simulink model "l512_devel_pps"  (R2012b)
settings: Solver=ode45  StartTime=0.0  StopTime=15000  RelTol=1e-3
undefined symbols (not defined in the file): sfp
libraries: xbsIndex_r4 x6414, casper_library_misc x268, casper_library_delays x134, xps_library x12, simulink x1, gavrt_library x1, xbsReplacements_r4 x1
(part 1 of 67)
settings Model: Creator=jkocz  LastModifiedBy=dprice
settings Model: ModifiedComment=|
  | dprice -- Mon Apr 06 20:09:48 2015 -- Version 1.459
  | Compiled successfully
settings Model: ModifiedHistory=|
  | dprice -- Mon Apr 06 20:09:48 2015 -- Version 1.459
  | Compiled successfully
  | 
  | dprice -- Mon Apr 06 16:18:15 2015 -- Version 1.458
  | 
  | Changed pps delay to about 0.1s
  | 
  | dprice -- Fri Mar 13 15:46:33 2015 -- Version 1.457
  | 
  | 
  | dprice -- Fri Mar 13 15:34:50 2015 -- Version 1.456
  | Copied triggering over to f1 - f4
  | 
  | dprice -- Fri Mar 13 15:31:03 2015 -- Version 1.455
  | 
  | Added better triggering of RMS monitor
  | 
  | dprice -- Wed Jan 21 17:17:07 2015 -- Version 1.454
  | 
  | 
  | dprice -- Wed Jan 21 14:02:39 2015 -- Version 1.453
  | changed to be triggered by correct pps
  | 
  | dprice -- Thu Jan 15 16:51:06 2015 -- Version 1.452
  | dropped core back to 200 MHz from 216 MHz
  | 
  | dprice -- Thu Jan 15 13:30:59 2015 -- Version 1.451
  | 
  | Changed to use PPS triggered vacc. Needs testing!
  | 
  | dprice -- Thu Jan 15 13:21:59 2015 -- Version 1.450
  | 
  | 
  | dprice -- Thu Jan 15 13:19:39 2015 -- Version 1.449
  | 
  | 
  | dprice -- Thu Jan 15 13:13:52 2015 -- Version 1.448
  | 
  | Adding pps triggered vacc
  | 
  | dprice -- Tue Jan 13 15:35:09 2015 -- Version 1.447
  | 
  | Updated to spectrometer f_engine core
  | 
  | dprice -- Wed Dec 17 17:14:12 2014 -- Version 1.446
  | 
  | added some snap blocks to do eq0 output rms tests
  | 
  | dprice -- Fri Nov 21 18:19:20 2014 -- Version 1.445
  | 
  | 
  | dprice -- Fri Nov 21 15:29:28 2014 -- Version 1.444
  | 
  | 
  | dprice -- Fri Nov 21 15:28:21 2014 -- Version 1.443
  | 
  | 
  | dprice -- Fri Nov 21 15:22:12 2014 -- Version 1.442
  | 
  | About to try a compile
  | 
  | dprice -- Fri Nov 21 15:19:27 2014 -- Version 1.441
  | 
  | 
  | dprice -- Fri Nov 21 15:10:28 2014 -- Version 1.440
  | 
  | about to crash :/
  | 
  | dprice -- Thu Dec 19 14:05:55 2013 -- Version 1.439
  | 
  | Removed scope blocks in 10GbE spacketizer
  | 
  | dprice -- Thu Dec 12 01:39:04 2013 -- Version 1.438
  | 
  | Moved pfb and eq to black boxes. Hopefully compile times are a little quicker now...
  | 
  | dprice -- Wed Dec 11 11:19:03 2013 -- Version 1.437
  | 
  | Updated coeff generator (cg) with separate sky BRAM for switching (sw_sky), renamed sky to bpass, and changed from 18 bit to 32 bit coefficients
  | 
  | dprice -- Tue Dec 10 14:55:05 2013 -- Version 1.436
  | 
  | Closing session
  | 
  | dprice -- Sat Dec 07 16:46:59 2013 -- Version 1.435
  | Fixed bool slicing on tgbe_en
  | 
  | dprice -- Wed Dec 04 22:02:25 2013 -- Version 1.434
  | 
  | Trying to compile with 4x gbes in the design
  | 
  | dprice -- Wed Dec 04 21:44:55 2013 -- Version 1.433
  | 
  | Added extra tgbe blocks for failover
  | 
  | dprice -- Wed Dec 04 17:45:31 2013 -- Version 1.432
  | 
  | Renamed coeff_gen cg to save on length of bram name
  | 
  | dprice -- Wed Dec 04 17:38:25 2013 -- Version 1.431
  | 
  | Copied logic across to all fft/fX blocks. Trying first compile.
  | 
  | dprice -- Wed Dec 04 17:29:39 2013 -- Version 1.430
  | 
  | Modified eq block to allow selecting between switched and all-sky modes
  | 
  | dprice -- Wed Dec 04 16:56:15 2013 -- Version 1.429
  | 
  | Adding switching assembly coefficient selection by pps
  | 
  | dprice -- Wed Nov 06 11:09:49 2013 -- Version 1.428
  | 
  | Changed back down to 216 MHz. Added a post-eq snap block for testing of equalization levels
  | 
  | dprice -- Tue Nov 05 18:21:00 2013 -- Version 1.427
  | 
  | Removed scopes as they bring up an irritating message each time you try and compile
  | 
  | dprice -- Tue Nov 05 14:30:34 2013 -- Version 1.426
  | 
  | Found timing issues with round block. Added a mask and increased latency in convert and multiply.
  | 
  | dprice -- Tue Nov 05 11:43:26 2013 -- Version 1.423
  | 
  | Changed clock to 239 MHz, just to see if it still compiles...
  | 
  | dprice -- Tue Nov 05 11:43:26 2013 -- Version 1.423
  | 
  | Changed clock to 239 MHz, just to see if it still compiles...
  | 
  | dprice -- Tue Nov 05 09:11:40 2013 -- Version 1.422
  | 
  | Design compiled successfully at 210 MHz using pblock constraints (hstack). Now bumping to 216 MHz.
  | Added status LEDs to design for PPS and TX
  | 
  | dprice -- Mon Nov 04 16:36:08 2013 -- Version 1.421
  | 
  | Added pipeline delays to yelllow block I/O in effort to aid timing. Worst offending net was the rst yellow block, presumably due to fanout.
  | 
  | Also modified the ADC thresholding logic to use a BRAM vector accumulator.
  | 
  | dprice -- Tue Oct 29 13:55:56 2013 -- Version 1.412
  | 
  | Fixed mux error - due to goto tag mismatch
  | 
  | dprice -- Tue Oct 29 13:55:56 2013 -- Version 1.412
  | 
  | Fixed mux error - due to goto tag mismatch
  | 
  | dprice -- Tue Oct 29 11:53:04 2013 -- Version 1.411
  | 
  | WTF is wrong with these mux blocks? Keep getting error on dtype in on muxes in packetbuffer.
  | 
  | dprice -- Mon Oct 28 18:12:23 2013 -- Version 1.410
  | 
  | 
  | dprice -- Mon Oct 28 18:11:25 2013 -- Version 1.409
  | 
  | Need to remove slice on FFT_SHIFTS
  | 
  | * Black boxed FFT
  | * Added ADC overflow logic and snap.
settings DataIOCC: SignalLoggingSaveFormat=ModelDataLogs
settings DebuggingCC: FcnCallInpInsideContextMsg=UseLocalSettings  StrictBusMsg=Warning
settings GRTTargetCC: CombineOutputUpdateFcns=off  GRTInterface=on

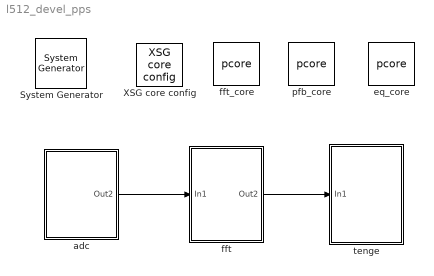
== system l512_devel_pps ==
  " System Generator" : xbsIndex_r4/ System Generator  Tag=genX  xilinxfamily=virtex6  part=xc6vsx475t  speed=-1  package=ff1759  synthesis_tool=XST  clock_wrapper=Clock Enables  directory=./l512_devel_pps/sysgen  proj_type=Project Navigator  Synth_file=XST Defaults  Impl_file=ISE Defaults  testbench=off  simulink_period=1  sysclk_period=5  dcm_input_clock_period=100  incr_netlist=off  trim_vbits=Everywhere in SubSystem  dbl_ovrd=According to Block Masks  core_generation=According to Block Masks  run_coregen=off  deprecated_control=off  eval_field=0  block_type=sysgen
      settings: block_version=11.4
  XSG core config : xps_library/XSG core config  Tag=xps:xsg  hw_sys=ROACH2:sx475t  clk_src=adc0_clk  ROACH_clk_src=adc0_clk  ROACH2_clk_src=adc0_clk  clk_rate=200  sample_period=1  synthesis_tool=XST
  adc : Subsystem
  eq_core : xps_library/pcore  Tag=xps:pcore  pcore_path=/data1/dprice/leda512/bb/eq_basic_core/eq_basic_core.ngc
  fft : Subsystem
  fft_core : xps_library/pcore  Tag=xps:pcore  pcore_path=/data1/dprice/leda512/bb/fft_core/fft_core.ngc
  pfb_core : xps_library/pcore  Tag=xps:pcore  pcore_path=/data1/dprice/leda512/bb/pfb_core/pfb_core.ngc
  tenge : Subsystem
  wires:
  adc/1(Out2) -> fft/1(In1)
  fft/1(Out2) -> tenge/1(In1)
